simulink model "sensors_actuators_dry_HIL"  (R2020a)
settings: Solver=FixedStepAuto  StartTime=0.0  StopTime=inf  RelTol=1e-3  EnableMultiTasking=on
undefined symbols (not defined in the file): standard
libraries: xpcutilitieslib x41, hdlsllib x24, simulink x7, slrtlib x4, xpcseriallib x2, speedgoatlib_IO581 x1
settings Model: SimulationMode=external  Creator=MAE-VermillionLab  LastModifiedBy=MAE-Vermillionlab
settings SolverCC: ConcurrentTasks=on  AutoInsertRateTranBlk=on
settings DataIOCC: SaveFormat=StructureWithTime
settings OptimizationCC: BlockReduction=off  OptimizeBlockIOStorage=off
settings HardwareCC: ProdBitPerPointer=32  ProdBitPerSizeT=32  ProdBitPerPtrDiffT=32  ProdLargestAtomicFloat=None  ProdWordSize=32  ProdLongLongMode=on  ProdHWDeviceType=Generic->32-bit x86 compatible
settings RTWCC: Description=Simulink Real-Time  SystemTargetFile=slrt.tlc  TemplateMakefile=slrt_default_tmf  CodeExecutionProfiling=on  RTWCompilerOptimization=on
settings SimulinkRealTimeCC: SupportVariableSizeSignals=on  RL32LogTETModifier=off  xPCConcurrentTasks=on

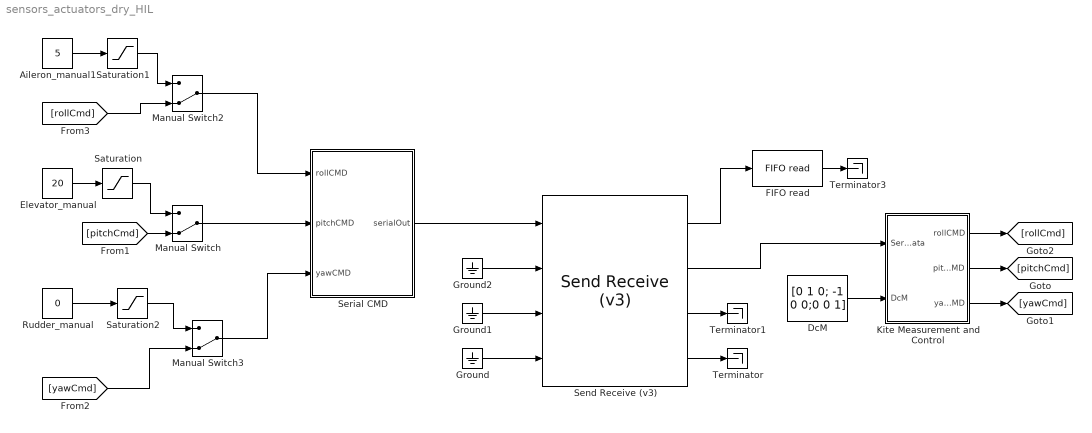
== system sensors_actuators_dry_HIL ==
  Aileron_manual1 : Constant  Value=5  OutDataTypeStr=int8
  DcM : Constant  Value=[0 1 0; -1 0 0;0 0 1]
  Elevator_manual : Constant  Value=20  OutDataTypeStr=int8
  "FIFO read " : xpcseriallib/FIFO read   maxsize=1024  minsize=1  usedelimiter=off  delimiter=13  outputtype=8 bit uint null terminated  enable=off  enableout=off  sampletime=.01
      settings: SourceProductBaseCode=XP
  Ground : Ground
  Ground1 : Ground
  Ground2 : Ground
  "Kite Measurement and Control " : Subsystem
  Manual Switch : ManualSwitch  CurrentSetting=0
  Manual Switch2 : ManualSwitch  CurrentSetting=0
  Manual Switch3 : ManualSwitch  CurrentSetting=0
  Rudder_manual : Constant  Value=0  OutDataTypeStr=int8
  Saturation : Saturate  UpperLimit=30  LowerLimit=-30
  Saturation1 : Saturate  UpperLimit=30  LowerLimit=-30
  Saturation2 : Saturate  UpperLimit=30  LowerLimit=-30
  "Send Receive (v3) " : speedgoatlib_IO581/Send Receive (v3)   parModuleId=1  parSlot=-1  parModuleType=IO581  parTransceiver12=RS485 Half-Duplex  parTransceiver34=RS232  parTransceiver1=RS485 Half-Duplex  parAutoTurnaround1=off  parTurnaroundDelay1=0  parStandardBaud1=on  parBaudrate1=115200  parBaudDivisor1=1  parSamplingRate1=16x (standard)  parPrescale1=off  parCalcBaud1=7812500  parParity1=None  parDataBits1=8  parStopBits1=1  parTxTrigLvl1=1  parRxTrigLvl1=1  parHandshake1=none  parRtsHysteresis1=0  parXon1=17  parXoff1=19  parTxSwFifoSize1=1024  parTxSwFifoType1=8 bit uint null terminated  parRxSwFifoSize1=1024  parTransceiver2=RS485 Half-Duplex  parAutoTurnaround2=off  parTurnaroundDelay2=0  parStandardBaud2=on  parBaudrate2=115200  parBaudDivisor2=1  parSamplingRate2=16x (standard)  parPrescale2=off  parCalcBaud2=7812500  parParity2=None  parDataBits2=8  parStopBits2=1  parTxTrigLvl2=1  parRxTrigLvl2=1  parHandshake2=none  parRtsHysteresis2=0  parXon2=17  parXoff2=19  parTxSwFifoSize2=1024  parTxSwFifoType2=8 bit int null terminated  parRxSwFifoSize2=1024  parTransceiver3=RS232  parAutoTurnaround3=off  parTurnaroundDelay3=0  parStandardBaud3=on  parBaudrate3=115200  parBaudDivisor3=1  parSamplingRate3=16x (standard)  parPrescale3=off  parCalcBaud3=7812500  parParity3=None  parDataBits3=8  parStopBits3=1  parTxTrigLvl3=1  parRxTrigLvl3=1  parHandshake3=none  parRtsHysteresis3=0  parXon3=17  parXoff3=19  parTxSwFifoSize3=1024  parTxSwFifoType3=8 bit uint null terminated  parRxSwFifoSize3=1024  parTransceiver4=RS232  parAutoTurnaround4=off  parTurnaroundDelay4=0  parStandardBaud4=on  parBaudrate4=115200  parBaudDivisor4=1  parSamplingRate4=16x (standard)  parPrescale4=off  parCalcBaud4=7812500  parParity4=None  parDataBits4=8  parStopBits4=1  parTxTrigLvl4=1  parRxTrigLvl4=1  parHandshake4=none  parRtsHysteresis4=0  parXon4=17  parXoff4=19  parTxSwFifoSize4=1024  parTxSwFifoType4=8 bit uint null terminated  parRxSwFifoSize4=1024
      settings: SourceProductName=Simulink Real-Time: Speedgoat Library
  Serial CMD : Subsystem
  Terminator : Terminator
  Terminator1 : Terminator
  Terminator3 : Terminator
  wires:
  "Send Receive (v3) "/1 -> "FIFO read "/1
  "Send Receive (v3) "/3 -> Terminator1/1
  "Send Receive (v3) "/4 -> Terminator/1
  Ground/1 -> "Send Receive (v3) "/4
  Ground2/1 -> "Send Receive (v3) "/2
  Ground1/1 -> "Send Receive (v3) "/3
  "Send Receive (v3) "/2 -> "Kite Measurement and Control "/1(SerialData)
  Serial CMD/1(serialOut) -> "Send Receive (v3) "/1
  "FIFO read "/1 -> Terminator3/1
  [pitchCmd] -> Manual Switch/2
  Elevator_manual/1 -> Saturation/1
  Saturation/1 -> Manual Switch/1
  Aileron_manual1/1 -> Saturation1/1
  Saturation1/1 -> Manual Switch2/1
  Saturation2/1 -> Manual Switch3/1
  Rudder_manual/1 -> Saturation2/1
  [rollCmd] -> Manual Switch2/2
  [yawCmd] -> Manual Switch3/2
  "Kite Measurement and Control "/3(yawCMD) -> [yawCmd]
  "Kite Measurement and Control "/2(pitchCMD) -> [pitchCmd]
  "Kite Measurement and Control "/1(rollCMD) -> [rollCmd]
  Manual Switch/1 -> Serial CMD/2(pitchCMD)
  Manual Switch2/1 -> Serial CMD/1("rollCMD ")
  Manual Switch3/1 -> Serial CMD/3(yawCMD)
  DcM/1 -> "Kite Measurement and Control "/2(DcM)

== system sensors_actuators_dry_HIL/Kite Measurement and Control  ==
  SerialData : Inport
  DcM : Inport  Port=2
  Bus Selector : BusSelector  OutputSignals=rollCmd,pitchCmd,yawCmd
  Controller1 : Subsystem  mask{ctrlSurfDefMax=45, pitchKP=1, yawKP=1, rollKP=1}
      mask prompts: ctrlSurfDefMax "Max Ctrlsurf def"; pitchKP "pitch Kp"; yawKP "yaw Kp"; rollKP "roll Kp"
  "Euler setpoints " : Subsystem  mask{EulerSP=[0 0 0]}
      mask prompts: EulerSP "Euler Setpoints"
  "Kite Measurements " : Subsystem
  rollCMD : Outport
  pitchCMD : Outport  Port=2
  yawCMD : Outport  Port=3
  wires:
  "Kite Measurements "/1(kiteMeasure) -> Controller1/2(kiteMeasure)  "kiteMeasure"
  "Euler setpoints "/1(setPoints) -> Controller1/1(setPoints)  "setPoints"
  Bus Selector/3 -> yawCMD/1  "<yawCmd>"
  Controller1/1(Cmd) -> Bus Selector/1
  Bus Selector/2 -> pitchCMD/1  "<pitchCmd>"
  Bus Selector/1 -> rollCMD/1  "<rollCmd>"
  SerialData/1 -> "Kite Measurements "/1(In1)
  DcM/1 -> "Kite Measurements "/2(Input)

== system sensors_actuators_dry_HIL/Serial CMD ==
  note: Subsystem
  "rollCMD " : Inport
  pitchCMD : Inport  Port=2
  yawCMD : Inport  Port=3
  Constant : Constant  Value=97  OutDataTypeStr=uint8
  Mux : Mux  Inputs=7
  Mux1 : Mux  Inputs=3
  Scope 1 : slrtlib/Displays and Logging/Scope   scopeno=3  scopetype=Target  autostart=on  viewmode=Graphical sliding  formatstr='%15.6f'  grid=on  ylimits=[-30,30]  nosamples=500  noprepostsamples=0  interleave=1  triggermode=FreeRun  triggersignal=1  trigsignalfromport=off  triggerlevel=0.0  triggerslope=Either  triggerscope=1  triggersample=0  filename=data.dat  mode=Lazy  writesize=512  autorestart=off  dynamicfilemode=off  maxwritefilesize=512*1024^2
  Scope 2 : slrtlib/Displays and Logging/Scope   scopeno=4  scopetype=Target  autostart=on  viewmode=Numerical  formatstr='%15.6f'  grid=on  ylimits=[0,100]  nosamples=500  noprepostsamples=0  interleave=1  triggermode=FreeRun  triggersignal=1  trigsignalfromport=off  triggerlevel=0.0  triggerslope=Either  triggerscope=1  triggersample=0  filename=data.dat  mode=Lazy  writesize=512  autorestart=off  dynamicfilemode=off  maxwritefilesize=512*1024^2
  deg-to-us : Subsystem
  deg-to-us1 : Subsystem
  deg-to-us2 : Subsystem
  to2uint1 : Subsystem
  to2uint2 : Subsystem
  to2uint8 : Subsystem
  serialOut : Outport
  wires:
  pitchCMD/1 -> Mux1/2, deg-to-us1/1(In1)  "pitchCMD"
  Constant/1 -> Mux/1
  to2uint8/1(Out1) -> Mux/2
  to2uint8/2(Out2) -> Mux/3
  yawCMD/1 -> Mux1/3, deg-to-us2/1(In1)  "yawCMD"
  Mux/1 -> Scope 2/1, serialOut/1
  Mux1/1 -> Scope 1/1
  "rollCMD "/1 -> Mux1/1, deg-to-us/1(In1)  "rollCMD"
  to2uint1/1(Out1) -> Mux/4
  to2uint1/2(Out2) -> Mux/5
  to2uint2/1(Out1) -> Mux/6
  to2uint2/2(Out2) -> Mux/7
  deg-to-us/1(Out1) -> to2uint8/1(" ")
  deg-to-us1/1(Out1) -> to2uint1/1(" ")
  deg-to-us2/1(Out1) -> to2uint2/1(" ")

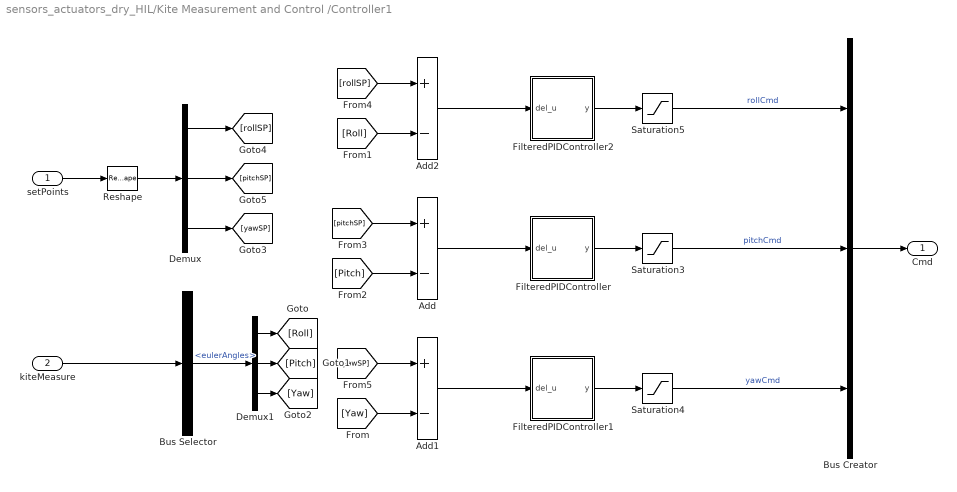
== system sensors_actuators_dry_HIL/Kite Measurement and Control /Controller1 ==
  setPoints : Inport
  kiteMeasure : Inport  Port=2
  Add : Sum  Inputs=+-
  Add1 : Sum  Inputs=+-
  Add2 : Sum  Inputs=+-
  Bus Creator : BusCreator  Inputs=3
  Bus Selector : BusSelector  OutputSignals=eulerAngles
  Demux : Demux  Outputs=3
  Demux1 : Demux  Outputs=3
  FilteredPIDController : Subsystem  mask{Kp=10, Kd=0, tau=0.01, Ki=0}
      mask prompts: Kp "Proportional Gain"; Kd "Derivative Gain"; tau "Time constant"; Ki "Integral Gain"
  FilteredPIDController1 : Subsystem  mask{Kp=10, Kd=0, tau=0.01, Ki=0}
      mask prompts: Kp "Proportional Gain"; Kd "Derivative Gain"; tau "Time constant"; Ki "Integral Gain"
  FilteredPIDController2 : Subsystem  mask{Kp=1, Kd=0, tau=0.01, Ki=0}
      mask prompts: Kp "Proportional Gain"; Kd "Derivative Gain"; tau "Time constant"; Ki "Integral Gain"
  Reshape : Reshape  OutputDimensionality=Column vector (2-D)
  Saturation3 : Saturate  UpperLimit=30  LowerLimit=-30
  Saturation4 : Saturate  UpperLimit=30  LowerLimit=-30
  Saturation5 : Saturate  UpperLimit=30  LowerLimit=-30
  Cmd : Outport
  wires:
  [Pitch] -> Add/2
  [Yaw] -> Add1/2
  [yawSP] -> Add1/1
  Demux/3 -> [yawSP]
  [pitchSP] -> Add/1
  kiteMeasure/1 -> Bus Selector/1
  Saturation3/1 -> Bus Creator/2  "pitchCmd"
  Saturation4/1 -> Bus Creator/3  "yawCmd"
  Saturation5/1 -> Bus Creator/1  "rollCmd"
  Bus Creator/1 -> Cmd/1
  Reshape/1 -> Demux/1
  setPoints/1 -> Reshape/1
  Add/1 -> FilteredPIDController/1(del_u)
  FilteredPIDController/1(y) -> Saturation3/1
  FilteredPIDController1/1(y) -> Saturation4/1
  Add1/1 -> FilteredPIDController1/1(del_u)
  FilteredPIDController2/1(y) -> Saturation5/1
  Add2/1 -> FilteredPIDController2/1(del_u)
  [rollSP] -> Add2/1
  [Roll] -> Add2/2
  Demux/2 -> [pitchSP]
  Demux/1 -> [rollSP]
  Bus Selector/1 -> Demux1/1  "<eulerAngles>"
  Demux1/1 -> [Roll]
  Demux1/2 -> [Pitch]
  Demux1/3 -> [Yaw]

== system sensors_actuators_dry_HIL/Kite Measurement and Control /Euler setpoints  ==
  Mux : Mux  Inputs=3
  Reshape : Reshape  OutputDimensionality=Column vector (2-D)
  pitchSP : Constant  Value=EulerSP(1)
  rollSP : Constant  Value=EulerSP(2)
  yawSP : Constant  Value=EulerSP(3)
  setPoints : Outport
  wires:
  rollSP/1 -> Mux/2  "rollSP"
  yawSP/1 -> Mux/3  "yawSP"
  pitchSP/1 -> Mux/1  "pitchSP"
  Mux/1 -> Reshape/1  "setPoints"
  Reshape/1 -> setPoints/1

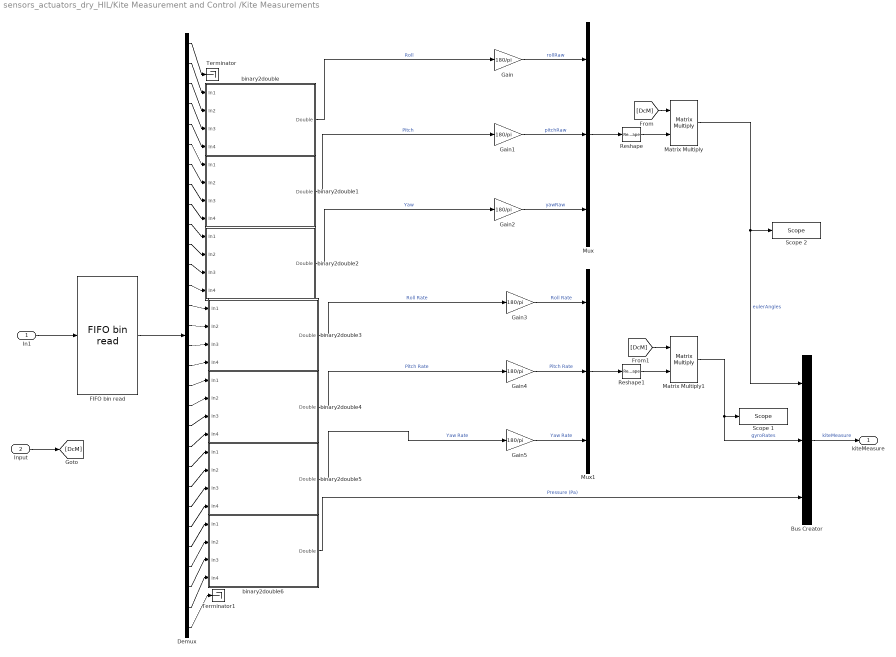
== system sensors_actuators_dry_HIL/Kite Measurement and Control /Kite Measurements  ==
  In1 : Inport
  Input : Inport  Port=2
  Bus Creator : BusCreator  Inputs=3
  Demux : Demux  Outputs=30
  "FIFO bin read " : xpcseriallib/FIFO bin read   header={[0x99]}  lengths=[29]  hold=Hold last output if no new data  enable=off  maxsize=29  outputtype=8 bit uint null terminated  sampletime=0.01
      settings: SourceProductBaseCode=XP
  Gain{,1..5} (6 alike) : Gain  Gain=180/pi
  Matrix Multiply : Product  Multiplication=Matrix(*)
  Matrix Multiply1 : Product  Multiplication=Matrix(*)
  Mux : Mux  Inputs=3
  Mux1 : Mux  Inputs=3
  Reshape : Reshape  OutputDimensionality=Column vector (2-D)
  Reshape1 : Reshape  OutputDimensionality=Column vector (2-D)
  Scope 1 : slrtlib/Displays and Logging/Scope   scopeno=2  scopetype=Target  autostart=on  viewmode=Graphical sliding  formatstr='%15.6f'  grid=on  ylimits=[-100,100]  nosamples=500  noprepostsamples=0  interleave=1  triggermode=FreeRun  triggersignal=1  trigsignalfromport=off  triggerlevel=0.0  triggerslope=Either  triggerscope=1  triggersample=0  filename=data.dat  mode=Lazy  writesize=512  autorestart=off  dynamicfilemode=off  maxwritefilesize=512*1024^2
  Scope 2 : slrtlib/Displays and Logging/Scope   scopeno=1  scopetype=Target  autostart=on  viewmode=Graphical sliding  formatstr='%15.6f'  grid=on  ylimits=[-100,100]  nosamples=500  noprepostsamples=0  interleave=1  triggermode=FreeRun  triggersignal=1  trigsignalfromport=off  triggerlevel=0.0  triggerslope=Either  triggerscope=1  triggersample=0  filename=data.dat  mode=Lazy  writesize=512  autorestart=off  dynamicfilemode=off  maxwritefilesize=512*1024^2
  Terminator : Terminator
  Terminator1 : Terminator
  binary2double : Subsystem
  binary2double1 : Subsystem
  binary2double2 : Subsystem
  binary2double3 : Subsystem
  binary2double4 : Subsystem
  binary2double5 : Subsystem
  binary2double6 : Subsystem
  kiteMeasure : Outport
  wires:
  binary2double/1(Double) -> Gain/1  "Roll"
  binary2double1/1(Double) -> Gain1/1  "Pitch"
  binary2double5/1(Double) -> Gain5/1  "Yaw Rate"
  binary2double6/1(Double) -> Bus Creator/3  "Pressure (Pa)"
  binary2double4/1(Double) -> Gain4/1  "Pitch Rate"
  binary2double3/1(Double) -> Gain3/1  "Roll Rate"
  binary2double2/1(Double) -> Gain2/1  "Yaw"
  Bus Creator/1 -> kiteMeasure/1  "kiteMeasure"
  Demux/25 -> binary2double5/4(In4)
  Demux/28 -> binary2double6/3(In3)
  Demux/10 -> binary2double2/1(In1)
  Demux/20 -> binary2double4/3(In3)
  Demux/18 -> binary2double4/1(In1)
  Demux/13 -> binary2double2/4(In4)
  Demux/30 -> Terminator1/1
  Demux/8 -> binary2double1/3(In3)
  Demux/19 -> binary2double4/2(In2)
  Demux/26 -> binary2double6/1(In1)
  Demux/16 -> binary2double3/3(In3)
  Demux/6 -> binary2double1/1(In1)
  Demux/4 -> binary2double/3(In3)
  In1/1 -> "FIFO bin read "/1
  Demux/7 -> binary2double1/2(In2)
  Demux/5 -> binary2double/4(In4)
  Demux/3 -> binary2double/2(In2)
  Demux/9 -> binary2double1/4(In4)
  Demux/11 -> binary2double2/2(In2)
  Demux/1 -> Terminator/1
  Demux/14 -> binary2double3/1(In1)
  Demux/15 -> binary2double3/2(In2)
  Demux/27 -> binary2double6/2(In2)
  Demux/22 -> binary2double5/1(In1)
  Demux/12 -> binary2double2/3(In3)
  Demux/2 -> binary2double/1(In1)
  Demux/23 -> binary2double5/2(In2)
  Demux/17 -> binary2double3/4(In4)
  Demux/29 -> binary2double6/4(In4)
  Demux/24 -> binary2double5/3(In3)
  Demux/21 -> binary2double4/4(In4)
  "FIFO bin read "/1 -> Demux/1
  Gain2/1 -> Mux/3  "yawRaw"
  Gain1/1 -> Mux/2  "pitchRaw"
  Gain/1 -> Mux/1  "rollRaw"
  Input/1 -> [DcM]
  Mux/1 -> Reshape/1
  Gain3/1 -> Mux1/1  "Roll Rate"
  Gain4/1 -> Mux1/2  "Pitch Rate"
  Gain5/1 -> Mux1/3  "Yaw Rate"
  Mux1/1 -> Reshape1/1
  Matrix Multiply/1 -> Scope 2/1, Bus Creator/1  "eulerAngles"
  Matrix Multiply1/1 -> Scope 1/1, Bus Creator/2  "gyroRates"
  Reshape/1 -> Matrix Multiply/2
  [DcM] -> Matrix Multiply/1
  Reshape1/1 -> Matrix Multiply1/2
  [DcM] -> Matrix Multiply1/1

== system sensors_actuators_dry_HIL/Serial CMD/deg-to-us ==
  In1 : Inport
  Constant1 : Constant  Value=1500
  Gain : Gain  Gain=1000/180
  Sum : Sum  Inputs=|++
  Out1 : Outport
  wires:
  Gain/1 -> Sum/1
  Constant1/1 -> Sum/2
  In1/1 -> Gain/1
  Sum/1 -> Out1/1

== system sensors_actuators_dry_HIL/Serial CMD/deg-to-us1 ==
  In1 : Inport
  Constant1 : Constant  Value=1500
  Gain : Gain  Gain=1000/180
  Sum : Sum  Inputs=|++
  Out1 : Outport
  wires:
  Sum/1 -> Out1/1
  In1/1 -> Gain/1
  Constant1/1 -> Sum/2
  Gain/1 -> Sum/1

== system sensors_actuators_dry_HIL/Serial CMD/deg-to-us2 ==
  In1 : Inport
  Constant1 : Constant  Value=1500
  Gain : Gain  Gain=1000/180
  Sum : Sum  Inputs=|++
  Out1 : Outport
  wires:
  Gain/1 -> Sum/1
  Constant1/1 -> Sum/2
  In1/1 -> Gain/1
  Sum/1 -> Out1/1

== system sensors_actuators_dry_HIL/Serial CMD/to2uint1 ==
  " " : Inport
  Bit Packing 1 : xpcutilitieslib/Bit Packing   MaskBitPatterns={[0:7]}  MaskPackDataType=uint8  MaskPackDataSize=[1]
      settings: SourceProductBaseCode=XP
  Bit Packing 2 : xpcutilitieslib/Bit Packing   MaskBitPatterns={[0:7]}  MaskPackDataType=uint8  MaskPackDataSize=[1]
      settings: SourceProductBaseCode=XP
  Bit Shift2 : hdlsllib/Logic and Bit Operations/Bit Shift  mode=Shift Right Arithmetic  N=8
  Cast4 : DataTypeConversion  OutDataTypeStr=uint16
  Out1 : Outport
  Out2 : Outport  Port=2
  wires:
  Bit Packing 1/1 -> Out1/1
  " "/1 -> Cast4/1
  Cast4/1 -> Bit Packing 1/1, Bit Shift2/1
  Bit Packing 2/1 -> Out2/1
  Bit Shift2/1 -> Bit Packing 2/1

== system sensors_actuators_dry_HIL/Serial CMD/to2uint2 ==
  " " : Inport
  Bit Packing 1 : xpcutilitieslib/Bit Packing   MaskBitPatterns={[0:7]}  MaskPackDataType=uint8  MaskPackDataSize=[1]
      settings: SourceProductBaseCode=XP
  Bit Packing 2 : xpcutilitieslib/Bit Packing   MaskBitPatterns={[0:7]}  MaskPackDataType=uint8  MaskPackDataSize=[1]
      settings: SourceProductBaseCode=XP
  Bit Shift2 : hdlsllib/Logic and Bit Operations/Bit Shift  mode=Shift Right Arithmetic  N=8
  Cast4 : DataTypeConversion  OutDataTypeStr=uint16
  Out1 : Outport
  Out2 : Outport  Port=2
  wires:
  Bit Shift2/1 -> Bit Packing 2/1
  Bit Packing 2/1 -> Out2/1
  Cast4/1 -> Bit Shift2/1, Bit Packing 1/1
  " "/1 -> Cast4/1
  Bit Packing 1/1 -> Out1/1

== system sensors_actuators_dry_HIL/Serial CMD/to2uint8 ==
  " " : Inport
  Bit Packing 1 : xpcutilitieslib/Bit Packing   MaskBitPatterns={[0:7]}  MaskPackDataType=uint8  MaskPackDataSize=[1]
      settings: SourceProductBaseCode=XP
  Bit Packing 2 : xpcutilitieslib/Bit Packing   MaskBitPatterns={[0:7]}  MaskPackDataType=uint8  MaskPackDataSize=[1]
      settings: SourceProductBaseCode=XP
  Bit Shift2 : hdlsllib/Logic and Bit Operations/Bit Shift  mode=Shift Right Arithmetic  N=8
  Cast4 : DataTypeConversion  OutDataTypeStr=uint16
  Out1 : Outport
  Out2 : Outport  Port=2
  wires:
  Bit Shift2/1 -> Bit Packing 2/1
  Cast4/1 -> Bit Shift2/1, Bit Packing 1/1
  " "/1 -> Cast4/1
  Bit Packing 1/1 -> Out1/1
  Bit Packing 2/1 -> Out2/1

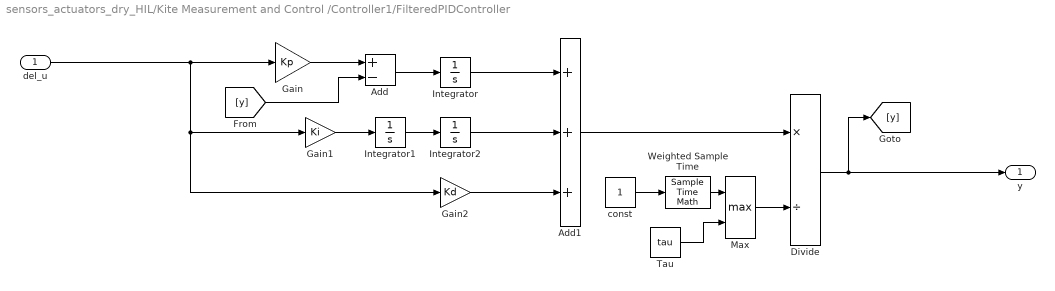
== system sensors_actuators_dry_HIL/Kite Measurement and Control /Controller1/FilteredPIDController ==
  del_u : Inport
  Add : Sum  Inputs=+-
  Add1 : Sum  Inputs=+++
  Divide : Product  Inputs=*/
  Gain : Gain  Gain=Kp
  Gain1 : Gain  Gain=Ki
  Gain2 : Gain  Gain=Kd
  Integrator : Integrator
  Integrator1 : Integrator
  Integrator2 : Integrator
  Max : MinMax  Function=max  Inputs=2
  Tau : Constant  Value=tau
  Weighted Sample Time : SampleTimeMath  TsampMathOp=Ts Only
  const : Constant
  y : Outport
  wires:
  Tau/1 -> Max/2
  del_u/1 -> Gain/1, Gain2/1, Gain1/1
  Divide/1 -> y/1, [y]
  Add/1 -> Integrator/1
  const/1 -> Weighted Sample Time/1
  Integrator/1 -> Add1/1
  Integrator1/1 -> Integrator2/1
  [y] -> Add/2
  Max/1 -> Divide/2
  Gain2/1 -> Add1/3
  Add1/1 -> Divide/1
  Gain1/1 -> Integrator1/1
  Gain/1 -> Add/1
  Weighted Sample Time/1 -> Max/1
  Integrator2/1 -> Add1/2

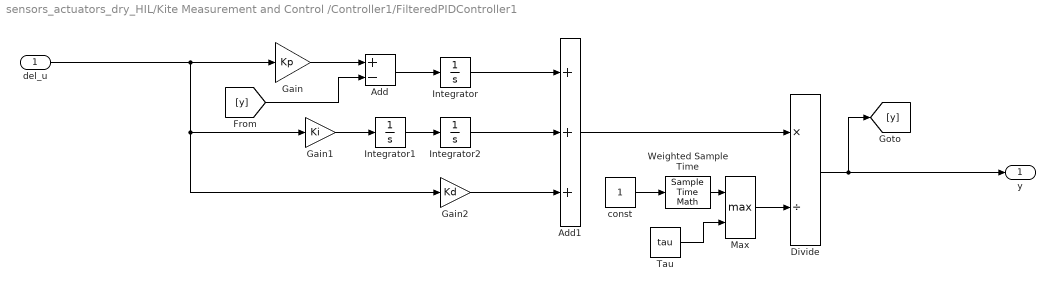
== system sensors_actuators_dry_HIL/Kite Measurement and Control /Controller1/FilteredPIDController1 ==
  del_u : Inport
  Add : Sum  Inputs=+-
  Add1 : Sum  Inputs=+++
  Divide : Product  Inputs=*/
  Gain : Gain  Gain=Kp
  Gain1 : Gain  Gain=Ki
  Gain2 : Gain  Gain=Kd
  Integrator : Integrator
  Integrator1 : Integrator
  Integrator2 : Integrator
  Max : MinMax  Function=max  Inputs=2
  Tau : Constant  Value=tau
  Weighted Sample Time : SampleTimeMath  TsampMathOp=Ts Only
  const : Constant
  y : Outport
  wires:
  Tau/1 -> Max/2
  del_u/1 -> Gain/1, Gain2/1, Gain1/1
  Divide/1 -> y/1, [y]
  Add/1 -> Integrator/1
  const/1 -> Weighted Sample Time/1
  Integrator/1 -> Add1/1
  Integrator1/1 -> Integrator2/1
  [y] -> Add/2
  Max/1 -> Divide/2
  Gain2/1 -> Add1/3
  Add1/1 -> Divide/1
  Gain1/1 -> Integrator1/1
  Gain/1 -> Add/1
  Weighted Sample Time/1 -> Max/1
  Integrator2/1 -> Add1/2

== system sensors_actuators_dry_HIL/Kite Measurement and Control /Controller1/FilteredPIDController2 ==
  del_u : Inport
  Add : Sum  Inputs=+-
  Add1 : Sum  Inputs=+++
  Divide : Product  Inputs=*/
  Gain : Gain  Gain=Kp
  Gain1 : Gain  Gain=Ki
  Gain2 : Gain  Gain=Kd
  Integrator : Integrator
  Integrator1 : Integrator
  Integrator2 : Integrator
  Max : MinMax  Function=max  Inputs=2
  Tau : Constant  Value=tau
  Weighted Sample Time : SampleTimeMath  TsampMathOp=Ts Only
  const : Constant
  y : Outport
  wires:
  Tau/1 -> Max/2
  del_u/1 -> Gain/1, Gain2/1, Gain1/1
  Divide/1 -> y/1, [y]
  Add/1 -> Integrator/1
  const/1 -> Weighted Sample Time/1
  Integrator/1 -> Add1/1
  Integrator1/1 -> Integrator2/1
  [y] -> Add/2
  Max/1 -> Divide/2
  Gain2/1 -> Add1/3
  Add1/1 -> Divide/1
  Gain1/1 -> Integrator1/1
  Gain/1 -> Add/1
  Weighted Sample Time/1 -> Max/1
  Integrator2/1 -> Add1/2

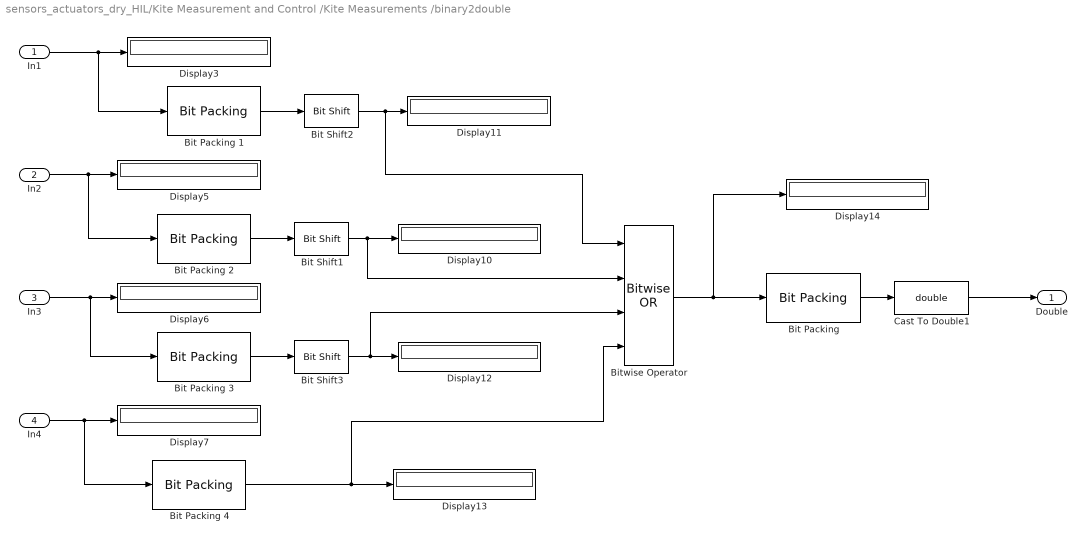
== system sensors_actuators_dry_HIL/Kite Measurement and Control /Kite Measurements /binary2double ==
  In1 : Inport
  In2 : Inport  Port=2
  In3 : Inport  Port=3
  In4 : Inport  Port=4
  Bit Packing {,1..4} (5 alike) : xpcutilitieslib/Bit Packing 
      settings: SourceProductBaseCode=XP
  Bit Shift1 : hdlsllib/Logic and Bit Operations/Bit Shift  mode=Shift Left Logical  N=16
  Bit Shift2 : hdlsllib/Logic and Bit Operations/Bit Shift  mode=Shift Left Logical  N=24
  Bit Shift3 : hdlsllib/Logic and Bit Operations/Bit Shift  mode=Shift Left Logical  N=8
  Bitwise Operator : simulink/Logic and Bit Operations/Bitwise Operator  logicop=OR  UseBitMask=off  NumInputPorts=4  BitMask=bin2dec('00000000')  BitMaskRealWorld=Stored Integer
  Cast To Double1 : DataTypeConversion  OutDataTypeStr=double
  Display{3,5..7,10..14} (9 alike) : Display
      settings: Format=hex (Stored Integer)
  Double : Outport
  wires:
  Bit Shift1/1 -> Bitwise Operator/2, Display10/1
  Bitwise Operator/1 -> Display14/1, "Bit Packing "/1
  Bit Packing 1/1 -> Bit Shift2/1
  Bit Packing 4/1 -> Bitwise Operator/4, Display13/1
  In1/1 -> Bit Packing 1/1, Display3/1
  In3/1 -> Bit Packing 3/1, Display6/1
  Bit Shift2/1 -> Bitwise Operator/1, Display11/1
  Bit Packing 2/1 -> Bit Shift1/1
  "Bit Packing "/1 -> Cast To Double1/1
  Bit Shift3/1 -> Bitwise Operator/3, Display12/1
  Bit Packing 3/1 -> Bit Shift3/1
  In2/1 -> Bit Packing 2/1, Display5/1
  In4/1 -> Bit Packing 4/1, Display7/1
  Cast To Double1/1 -> Double/1

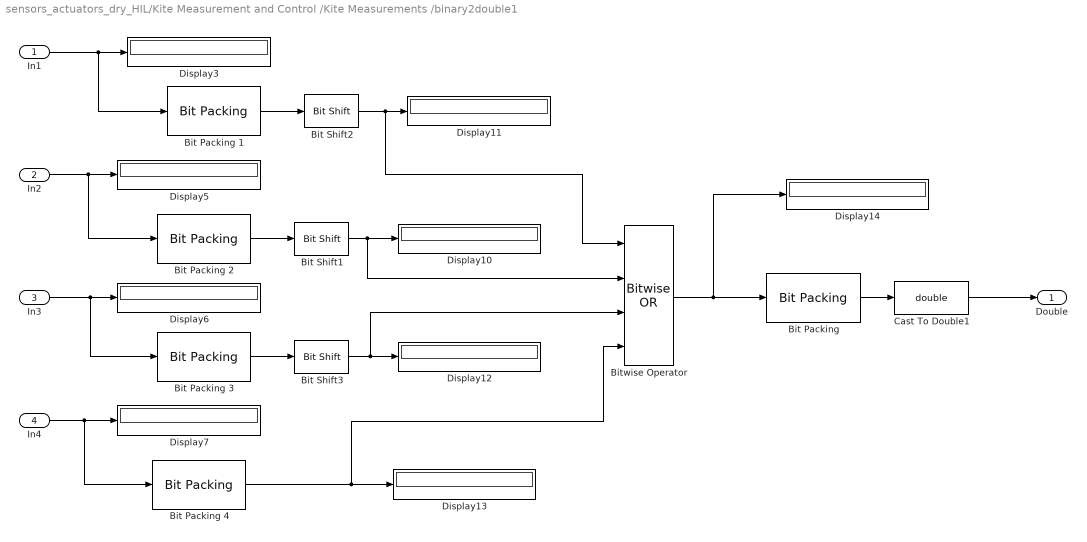
== system sensors_actuators_dry_HIL/Kite Measurement and Control /Kite Measurements /binary2double1 ==
  In1 : Inport
  In2 : Inport  Port=2
  In3 : Inport  Port=3
  In4 : Inport  Port=4
  Bit Packing {,1..4} (5 alike) : xpcutilitieslib/Bit Packing 
      settings: SourceProductBaseCode=XP
  Bit Shift1 : hdlsllib/Logic and Bit Operations/Bit Shift  mode=Shift Left Logical  N=16
  Bit Shift2 : hdlsllib/Logic and Bit Operations/Bit Shift  mode=Shift Left Logical  N=24
  Bit Shift3 : hdlsllib/Logic and Bit Operations/Bit Shift  mode=Shift Left Logical  N=8
  Bitwise Operator : simulink/Logic and Bit Operations/Bitwise Operator  logicop=OR  UseBitMask=off  NumInputPorts=4  BitMask=bin2dec('00000000')  BitMaskRealWorld=Stored Integer
  Cast To Double1 : DataTypeConversion  OutDataTypeStr=double
  Display{3,5..7,10..14} (9 alike) : Display
      settings: Format=hex (Stored Integer)
  Double : Outport
  wires:
  Bit Shift1/1 -> Bitwise Operator/2, Display10/1
  Bitwise Operator/1 -> Display14/1, "Bit Packing "/1
  Bit Packing 1/1 -> Bit Shift2/1
  Bit Packing 4/1 -> Bitwise Operator/4, Display13/1
  In1/1 -> Bit Packing 1/1, Display3/1
  In3/1 -> Bit Packing 3/1, Display6/1
  Bit Shift2/1 -> Bitwise Operator/1, Display11/1
  Bit Packing 2/1 -> Bit Shift1/1
  "Bit Packing "/1 -> Cast To Double1/1
  Bit Shift3/1 -> Bitwise Operator/3, Display12/1
  Bit Packing 3/1 -> Bit Shift3/1
  In2/1 -> Bit Packing 2/1, Display5/1
  In4/1 -> Bit Packing 4/1, Display7/1
  Cast To Double1/1 -> Double/1

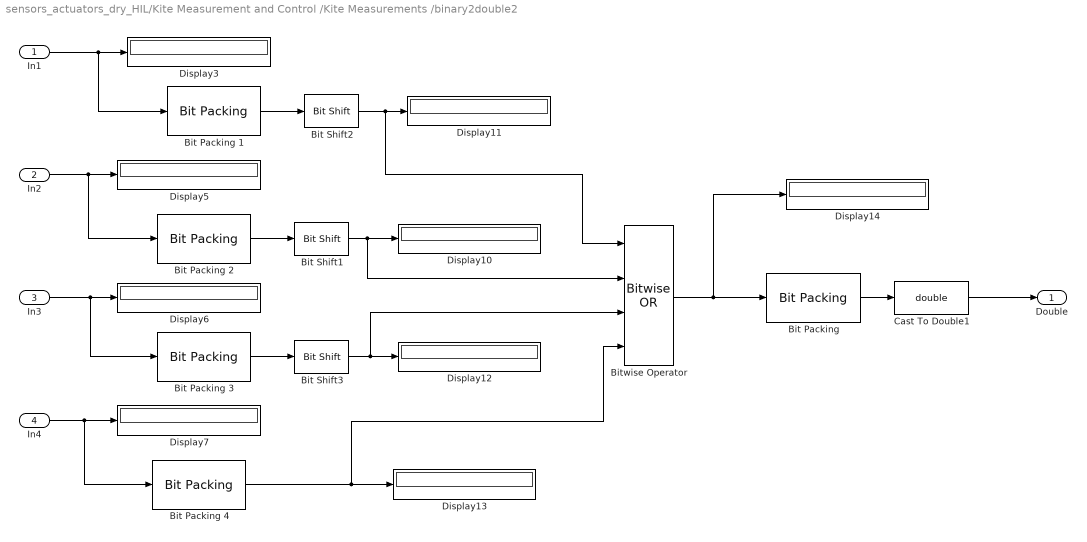
== system sensors_actuators_dry_HIL/Kite Measurement and Control /Kite Measurements /binary2double2 ==
  In1 : Inport
  In2 : Inport  Port=2
  In3 : Inport  Port=3
  In4 : Inport  Port=4
  Bit Packing {,1..4} (5 alike) : xpcutilitieslib/Bit Packing 
      settings: SourceProductBaseCode=XP
  Bit Shift1 : hdlsllib/Logic and Bit Operations/Bit Shift  mode=Shift Left Logical  N=16
  Bit Shift2 : hdlsllib/Logic and Bit Operations/Bit Shift  mode=Shift Left Logical  N=24
  Bit Shift3 : hdlsllib/Logic and Bit Operations/Bit Shift  mode=Shift Left Logical  N=8
  Bitwise Operator : simulink/Logic and Bit Operations/Bitwise Operator  logicop=OR  UseBitMask=off  NumInputPorts=4  BitMask=bin2dec('00000000')  BitMaskRealWorld=Stored Integer
  Cast To Double1 : DataTypeConversion  OutDataTypeStr=double
  Display{3,5..7,10..14} (9 alike) : Display
      settings: Format=hex (Stored Integer)
  Double : Outport
  wires:
  Bit Shift1/1 -> Bitwise Operator/2, Display10/1
  Bitwise Operator/1 -> Display14/1, "Bit Packing "/1
  Bit Packing 1/1 -> Bit Shift2/1
  Bit Packing 4/1 -> Bitwise Operator/4, Display13/1
  In1/1 -> Bit Packing 1/1, Display3/1
  In3/1 -> Bit Packing 3/1, Display6/1
  Bit Shift2/1 -> Bitwise Operator/1, Display11/1
  Bit Packing 2/1 -> Bit Shift1/1
  "Bit Packing "/1 -> Cast To Double1/1
  Bit Shift3/1 -> Bitwise Operator/3, Display12/1
  Bit Packing 3/1 -> Bit Shift3/1
  In2/1 -> Bit Packing 2/1, Display5/1
  In4/1 -> Bit Packing 4/1, Display7/1
  Cast To Double1/1 -> Double/1

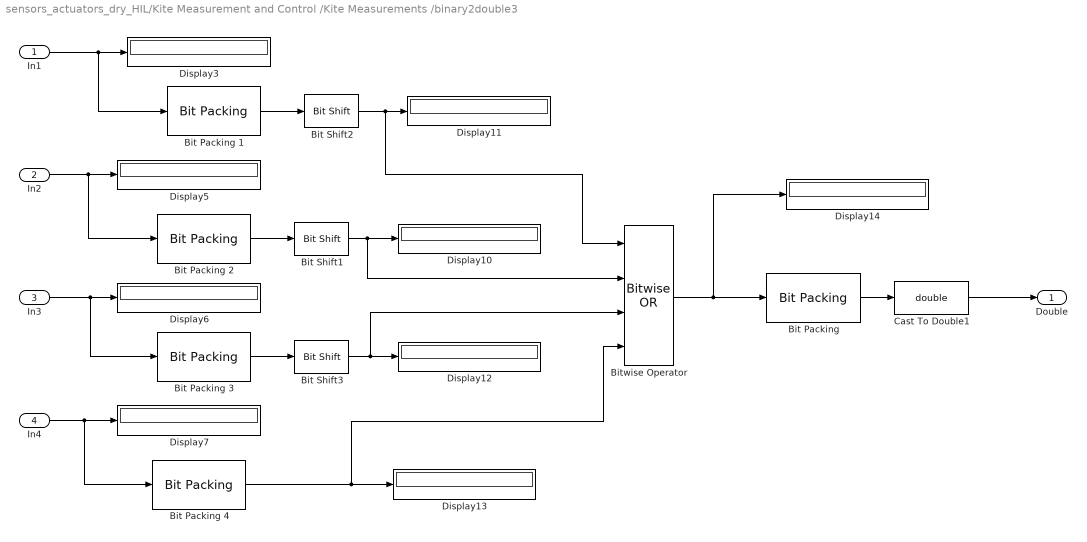
== system sensors_actuators_dry_HIL/Kite Measurement and Control /Kite Measurements /binary2double3 ==
  In1 : Inport
  In2 : Inport  Port=2
  In3 : Inport  Port=3
  In4 : Inport  Port=4
  Bit Packing {,1..4} (5 alike) : xpcutilitieslib/Bit Packing 
      settings: SourceProductBaseCode=XP
  Bit Shift1 : hdlsllib/Logic and Bit Operations/Bit Shift  mode=Shift Left Logical  N=16
  Bit Shift2 : hdlsllib/Logic and Bit Operations/Bit Shift  mode=Shift Left Logical  N=24
  Bit Shift3 : hdlsllib/Logic and Bit Operations/Bit Shift  mode=Shift Left Logical  N=8
  Bitwise Operator : simulink/Logic and Bit Operations/Bitwise Operator  logicop=OR  UseBitMask=off  NumInputPorts=4  BitMask=bin2dec('00000000')  BitMaskRealWorld=Stored Integer
  Cast To Double1 : DataTypeConversion  OutDataTypeStr=double
  Display{3,5..7,10..14} (9 alike) : Display
      settings: Format=hex (Stored Integer)
  Double : Outport
  wires:
  Bit Shift1/1 -> Bitwise Operator/2, Display10/1
  Bitwise Operator/1 -> Display14/1, "Bit Packing "/1
  Bit Packing 1/1 -> Bit Shift2/1
  Bit Packing 4/1 -> Bitwise Operator/4, Display13/1
  In1/1 -> Bit Packing 1/1, Display3/1
  In3/1 -> Bit Packing 3/1, Display6/1
  Bit Shift2/1 -> Bitwise Operator/1, Display11/1
  Bit Packing 2/1 -> Bit Shift1/1
  "Bit Packing "/1 -> Cast To Double1/1
  Bit Shift3/1 -> Bitwise Operator/3, Display12/1
  Bit Packing 3/1 -> Bit Shift3/1
  In2/1 -> Bit Packing 2/1, Display5/1
  In4/1 -> Bit Packing 4/1, Display7/1
  Cast To Double1/1 -> Double/1

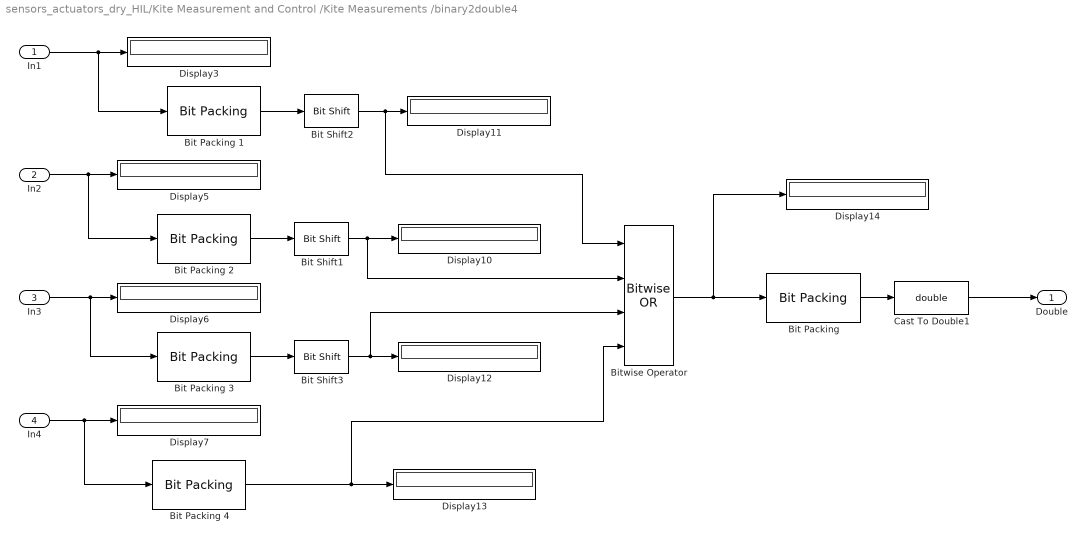
== system sensors_actuators_dry_HIL/Kite Measurement and Control /Kite Measurements /binary2double4 ==
  In1 : Inport
  In2 : Inport  Port=2
  In3 : Inport  Port=3
  In4 : Inport  Port=4
  Bit Packing {,1..4} (5 alike) : xpcutilitieslib/Bit Packing 
      settings: SourceProductBaseCode=XP
  Bit Shift1 : hdlsllib/Logic and Bit Operations/Bit Shift  mode=Shift Left Logical  N=16
  Bit Shift2 : hdlsllib/Logic and Bit Operations/Bit Shift  mode=Shift Left Logical  N=24
  Bit Shift3 : hdlsllib/Logic and Bit Operations/Bit Shift  mode=Shift Left Logical  N=8
  Bitwise Operator : simulink/Logic and Bit Operations/Bitwise Operator  logicop=OR  UseBitMask=off  NumInputPorts=4  BitMask=bin2dec('00000000')  BitMaskRealWorld=Stored Integer
  Cast To Double1 : DataTypeConversion  OutDataTypeStr=double
  Display{3,5..7,10..14} (9 alike) : Display
      settings: Format=hex (Stored Integer)
  Double : Outport
  wires:
  Bit Shift1/1 -> Bitwise Operator/2, Display10/1
  Bitwise Operator/1 -> Display14/1, "Bit Packing "/1
  Bit Packing 1/1 -> Bit Shift2/1
  Bit Packing 4/1 -> Bitwise Operator/4, Display13/1
  In1/1 -> Bit Packing 1/1, Display3/1
  In3/1 -> Bit Packing 3/1, Display6/1
  Bit Shift2/1 -> Bitwise Operator/1, Display11/1
  Bit Packing 2/1 -> Bit Shift1/1
  "Bit Packing "/1 -> Cast To Double1/1
  Bit Shift3/1 -> Bitwise Operator/3, Display12/1
  Bit Packing 3/1 -> Bit Shift3/1
  In2/1 -> Bit Packing 2/1, Display5/1
  In4/1 -> Bit Packing 4/1, Display7/1
  Cast To Double1/1 -> Double/1

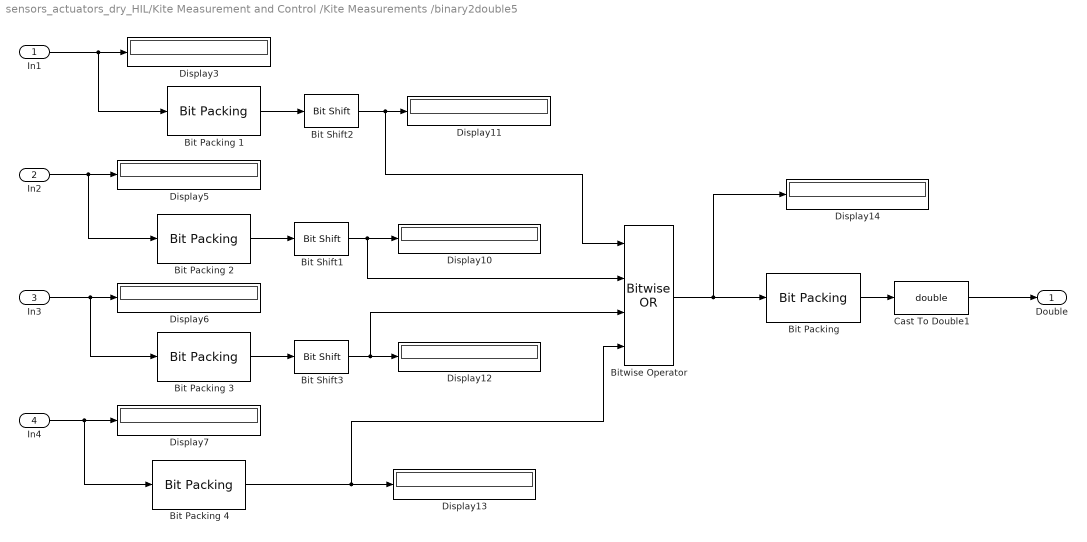
== system sensors_actuators_dry_HIL/Kite Measurement and Control /Kite Measurements /binary2double5 ==
  In1 : Inport
  In2 : Inport  Port=2
  In3 : Inport  Port=3
  In4 : Inport  Port=4
  Bit Packing {,1..4} (5 alike) : xpcutilitieslib/Bit Packing 
      settings: SourceProductBaseCode=XP
  Bit Shift1 : hdlsllib/Logic and Bit Operations/Bit Shift  mode=Shift Left Logical  N=16
  Bit Shift2 : hdlsllib/Logic and Bit Operations/Bit Shift  mode=Shift Left Logical  N=24
  Bit Shift3 : hdlsllib/Logic and Bit Operations/Bit Shift  mode=Shift Left Logical  N=8
  Bitwise Operator : simulink/Logic and Bit Operations/Bitwise Operator  logicop=OR  UseBitMask=off  NumInputPorts=4  BitMask=bin2dec('00000000')  BitMaskRealWorld=Stored Integer
  Cast To Double1 : DataTypeConversion  OutDataTypeStr=double
  Display{3,5..7,10..14} (9 alike) : Display
      settings: Format=hex (Stored Integer)
  Double : Outport
  wires:
  Bit Shift1/1 -> Bitwise Operator/2, Display10/1
  Bitwise Operator/1 -> Display14/1, "Bit Packing "/1
  Bit Packing 1/1 -> Bit Shift2/1
  Bit Packing 4/1 -> Bitwise Operator/4, Display13/1
  In1/1 -> Bit Packing 1/1, Display3/1
  In3/1 -> Bit Packing 3/1, Display6/1
  Bit Shift2/1 -> Bitwise Operator/1, Display11/1
  Bit Packing 2/1 -> Bit Shift1/1
  "Bit Packing "/1 -> Cast To Double1/1
  Bit Shift3/1 -> Bitwise Operator/3, Display12/1
  Bit Packing 3/1 -> Bit Shift3/1
  In2/1 -> Bit Packing 2/1, Display5/1
  In4/1 -> Bit Packing 4/1, Display7/1
  Cast To Double1/1 -> Double/1

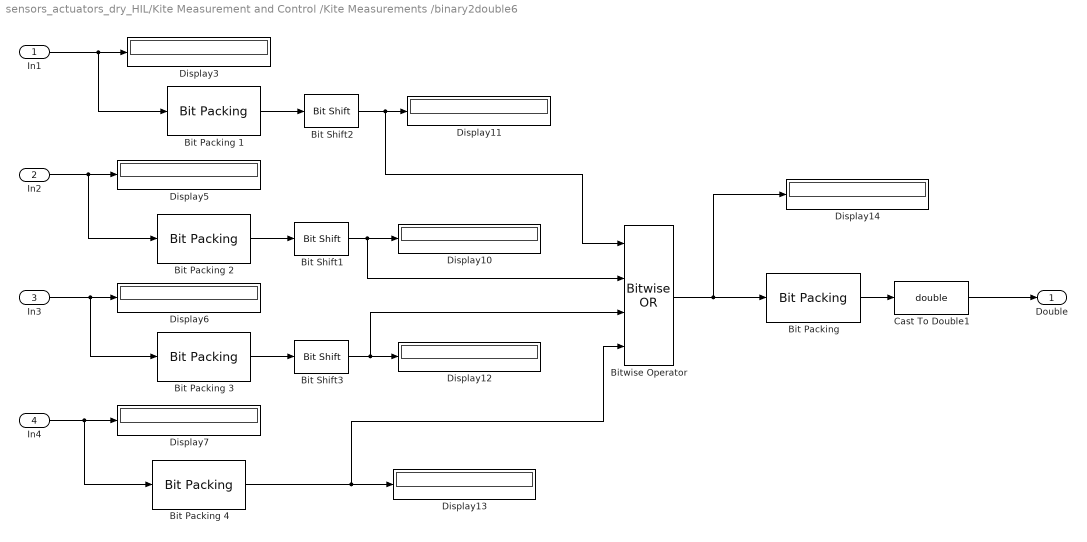
== system sensors_actuators_dry_HIL/Kite Measurement and Control /Kite Measurements /binary2double6 ==
  In1 : Inport
  In2 : Inport  Port=2
  In3 : Inport  Port=3
  In4 : Inport  Port=4
  Bit Packing {,1..4} (5 alike) : xpcutilitieslib/Bit Packing 
      settings: SourceProductBaseCode=XP
  Bit Shift1 : hdlsllib/Logic and Bit Operations/Bit Shift  mode=Shift Left Logical  N=16
  Bit Shift2 : hdlsllib/Logic and Bit Operations/Bit Shift  mode=Shift Left Logical  N=24
  Bit Shift3 : hdlsllib/Logic and Bit Operations/Bit Shift  mode=Shift Left Logical  N=8
  Bitwise Operator : simulink/Logic and Bit Operations/Bitwise Operator  logicop=OR  UseBitMask=off  NumInputPorts=4  BitMask=bin2dec('00000000')  BitMaskRealWorld=Stored Integer
  Cast To Double1 : DataTypeConversion  OutDataTypeStr=double
  Display{3,5..7,10..14} (9 alike) : Display
      settings: Format=hex (Stored Integer)
  Double : Outport
  wires:
  Bit Shift1/1 -> Bitwise Operator/2, Display10/1
  Bitwise Operator/1 -> Display14/1, "Bit Packing "/1
  Bit Packing 1/1 -> Bit Shift2/1
  Bit Packing 4/1 -> Bitwise Operator/4, Display13/1
  In1/1 -> Bit Packing 1/1, Display3/1
  In3/1 -> Bit Packing 3/1, Display6/1
  Bit Shift2/1 -> Bitwise Operator/1, Display11/1
  Bit Packing 2/1 -> Bit Shift1/1
  "Bit Packing "/1 -> Cast To Double1/1
  Bit Shift3/1 -> Bitwise Operator/3, Display12/1
  Bit Packing 3/1 -> Bit Shift3/1
  In2/1 -> Bit Packing 2/1, Display5/1
  In4/1 -> Bit Packing 4/1, Display7/1
  Cast To Double1/1 -> Double/1
